simulink model "finalll"  (R2016b)
settings: Solver=FixedStepDiscrete  StartTime=0.0  StopTime=10.0  RelTol=1e-3
settings Model: Creator=Radwa  LastModifiedBy=Radwa
settings SolverCC: EnableConcurrentExecution=on
settings DataIOCC: ReturnWorkspaceOutputs=on
settings OptimizationCC: DefaultParameterBehavior=Inlined  EnhancedBackFolding=on  PassReuseOutputArgsAs=Individual arguments
settings DebuggingCC: ParameterTunabilityLossMsg=error
settings SFSimCC: SimUseLocalCustomCode=on
settings RTWCC: SystemTargetFile=ert.tlc  GenCodeOnly=on  TemplateMakefile=ert_default_tmf  Description=Embedded Coder  GenerateReport=on  RTWUseLocalCustomCode=on  IncludeHyperlinkInReport=on  LaunchReport=on  GenerateTraceInfo=on  GenerateTraceReport=on  GenerateTraceReportSl=on  GenerateTraceReportSf=on  GenerateTraceReportEml=on
settings CodeAppCC: ForceParamTrailComments=on  IgnoreCustomStorageClasses=off  OperatorAnnotations=on  SimulinkDataObjDesc=on  SFDataObjDesc=on  InsertBlockDesc=on
settings ERTTargetCC: TargetLangStandard=C99 (ISO)  MultiwordLength=256  GenerateSampleERTMain=on  InlinedParameterPlacement=NonHierarchical  ERTCustomFileTemplate=example_file_process.tlc

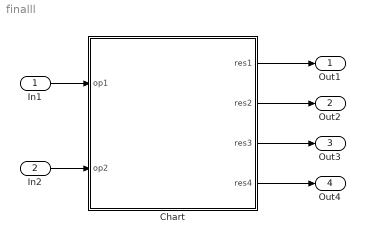
== system finalll ==
  In1 : Inport
  In2 : Inport  Port=2
  Chart : Stateflow chart  TreatAsAtomicUnit=on
  Out1 : Outport
  Out2 : Outport  Port=2
  Out3 : Outport  Port=3
  Out4 : Outport  Port=4
  wires:
  In1/1 -> Chart/1(op1)
  In2/1 -> Chart/2(op2)
  Chart/1(res1) -> Out1/1
  Chart/2(res2) -> Out2/1
  Chart/3(res3) -> Out3/1
  Chart/4(res4) -> Out4/1

== stateflow chart finalll/Chart ==
  state addRes  = Add(  num1, num2) [function]
    (default) -> (junction 8) : {addRes= num1+num2;}
  state subRes  = Sub(  num1, num2) [function]
    (default) -> (junction 42) : {subRes= num1-num2;}
  state mulRes  = Mul(  num1, num2) [function]
    (default) -> (junction 48) : {mulRes= num1*num2;}
  state divRes  = Div(  num1, num2) [function]
    (default) -> (junction 54) : {divRes= num1/num2;}
  (default) -> (junction 18)
  (junction 18) -> (junction 25) : {res1=Add(op1,op2);
      | res2=Sub(op1,op2);
      | res3=Mul(op1,op2);
      | res4=Div(op1,op2);
      | }
  data: num1 function_input uint32 size=1; num2 function_input uint32 size=1; addRes function_output uint32 size=1; num1 function_input uint32 size=1; num2 function_input uint32 size=1; subRes function_output uint32 size=1; num1 function_input uint32 size=1; num2 function_input uint32 size=1; mulRes function_output uint32 size=1; num1 function_input uint32 size=1; num2 function_input uint32 size=1; divRes function_output uint32 size=1; res1 output uint32 size=1; op1 input uint32 size=1; op2 input uint32 size=1; res2 output uint32 size=1; res3 output uint32 size=1; res4 output uint32 size=1
